simulink model "prefilter"  (R2015b)
settings: Solver=FixedStepDiscrete  StartTime=0.0  StopTime=10.0  FixedStep=10e-3  RelTol=1e-3
InitFcn:
  | initialization
undefined symbols (not defined in the file): Amax, Amin, DiscIntNeverNeededParam, Tau, Ts_Filter, V0, Vmax, Vmin, X0, Xmax, Xmin
libraries: simulink x3, simulink_extras x1
settings Model: Creator=valentin_riviere  LastModifiedBy=valentin_riviere

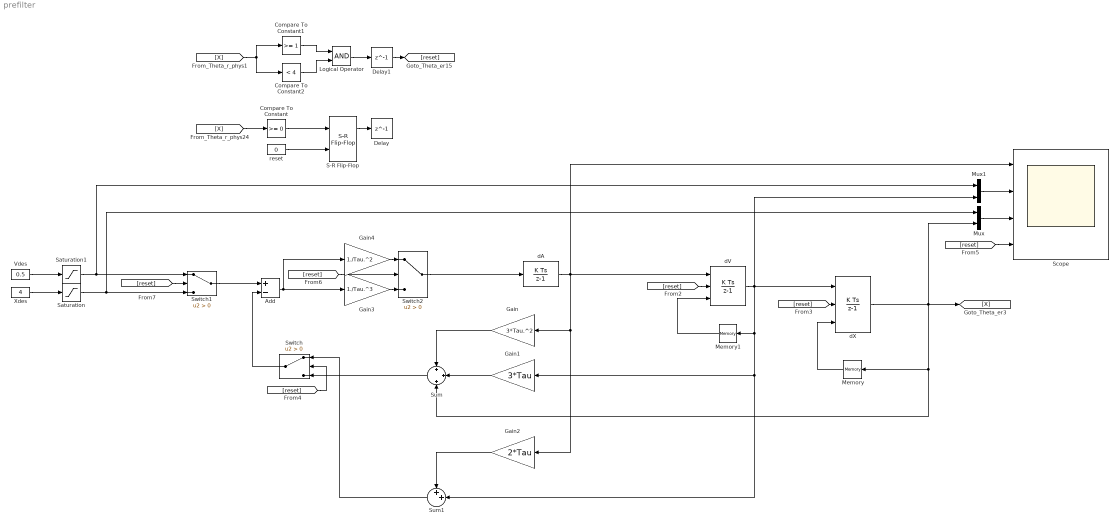
== system prefilter ==
  Add : Sum  Inputs=+-
  Compare To Constant : simulink/Logic and Bit Operations/Compare To Constant  relop=>=  const=0  OutDataTypeStr=boolean
  Compare To Constant1 : simulink/Logic and Bit Operations/Compare To Constant  relop=>=  const=1  OutDataTypeStr=boolean
  Compare To Constant2 : simulink/Logic and Bit Operations/Compare To Constant  relop=<  const=4  OutDataTypeStr=boolean
  Delay : Delay  DelayLength=1  InitialCondition=0
  Delay1 : Delay  DelayLength=1  InitialCondition=0
  Gain : Gain  Gain=3*Tau.^2
  Gain1 : Gain  Gain=3*Tau
  Gain2 : Gain  Gain=2*Tau
  Gain3 : Gain  Gain=1./Tau.^3
  Gain4 : Gain  Gain=1./Tau.^2
  Logical Operator : Logic  AllPortsSameDT=off  OutDataTypeStr=boolean
  Memory : Memory  X0=X0  InheritSampleTime=on
  Memory1 : Memory  X0=V0  InheritSampleTime=on
  Mux : Mux  Inputs=2
  Mux1 : Mux  Inputs=2
  S-R Flip-Flop : simulink_extras/Flip Flops/S-R Flip-Flop  initial_condition=0
  Saturation : Saturate  UpperLimit=Xmax  LowerLimit=Xmin
  Saturation1 : Saturate  UpperLimit=Vmax  LowerLimit=Vmin
  Scope : Scope  NumInputPorts=4
  Sum : Sum  Inputs=+|+|+
  Sum1 : Sum  Inputs=++|
  Switch : Switch  Criteria=u2 > Threshold
  Switch1 : Switch  Criteria=u2 > Threshold
  Switch2 : Switch  Criteria=u2 > Threshold
  Vdes : Constant  Value=0.5  SampleTime=-1
  Xdes : Constant  Value=4  SampleTime=-1
  dA : DiscreteIntegrator  SampleTime=Ts_Filter  LimitOutput=on  UpperSaturationLimit=Amax  LowerSaturationLimit=Amin  ICPrevOutput=DiscIntNeverNeededParam  ICPrevScaledInput=DiscIntNeverNeededParam
  dV : DiscreteIntegrator  ExternalReset=either  InitialConditionSource=external  SampleTime=Ts_Filter  LimitOutput=on  UpperSaturationLimit=Vmax  LowerSaturationLimit=Vmin  ICPrevOutput=DiscIntNeverNeededParam  ICPrevScaledInput=DiscIntNeverNeededParam
  dX : DiscreteIntegrator  ExternalReset=either  InitialConditionSource=external  SampleTime=Ts_Filter  LimitOutput=on  UpperSaturationLimit=Xmax  LowerSaturationLimit=Xmin  ICPrevOutput=DiscIntNeverNeededParam  ICPrevScaledInput=DiscIntNeverNeededParam
  reset : Constant  Value=0  OutDataTypeStr=Inherit: Inherit via back propagation  SampleTime=-1
  wires:
  Saturation/1 -> Switch1/3, Mux/1
  Switch2/1 -> dA/1
  Gain/1 -> Sum/1
  Gain1/1 -> Sum/2
  dA/1 -> Gain2/1, Gain/1, dV/1, Scope/1
  dX/1 -> Sum/3, Memory/1, Mux/2, [X]
  Memory1/1 -> dV/3
  Xdes/1 -> Saturation/1
  Mux/1 -> Scope/3
  [X] -> Compare To Constant/1
  Memory/1 -> dX/3
  Compare To Constant/1 -> S-R Flip-Flop/1
  Switch1/1 -> Add/1
  Vdes/1 -> Saturation1/1
  Saturation1/1 -> Mux1/1, Switch1/1
  Mux1/1 -> Scope/2
  S-R Flip-Flop/1 -> Delay/1
  reset/1 -> S-R Flip-Flop/2
  [reset] -> Switch1/2
  [reset] -> dV/2
  [reset] -> dX/2
  [reset] -> Scope/4
  [reset] -> Switch/2
  Sum/1 -> Switch/3
  Switch/1 -> Add/2
  Sum1/1 -> Switch/1
  dV/1 -> Sum1/2, Gain1/1, Memory1/1, Mux1/2, dX/1
  Gain2/1 -> Sum1/1
  Add/1 -> Gain4/1, Gain3/1
  [reset] -> Switch2/2
  Gain3/1 -> Switch2/3
  Gain4/1 -> Switch2/1
  Delay1/1 -> [reset]
  [X] -> Compare To Constant1/1, Compare To Constant2/1
  Logical Operator/1 -> Delay1/1
  Compare To Constant1/1 -> Logical Operator/1
  Compare To Constant2/1 -> Logical Operator/2
